simulink model "X8_demo"  (R2015b)
settings: Solver=ode45  StartTime=0.0  StopTime=150  RelTol=1e-3
values from neighbouring files (symbols this model uses):
  end_time = 150    [initX8_demo.m]
  h_ref = 100    [init.m]    (also in initX8_demo.m)
  input_source = 3    [initX8_demo.m]    (also in runX8.m)
  input_source0 = 1    [initX8_demo.m]    (also in runX8.m)
  input_step_time = 0    [initX8_demo.m]    (also in runX8.m = 2)
  lat0 = 37.6205    [init.m]    (also in initX8_demo.m)
  lon0 = -122.3815    [init.m]    (also in initX8_demo.m)
  U_trim = [0.0079    0.0000         0    0.1240]'    [initX8_demo.m]    (also in runX8.m = [0.0079    0.0000         0    0.1240])
  X_trim = [0.0000    0.0000 -150.0000    0.9997    0.0000    0.0232   -0.0000 18.0168    0.0001    0.8366    0.0000    0.0000    0.0000 0.0039 -0.0000    0.0039   -0.0000    0.1240]'    [initX8_demo.m]    (also in runX8.m = x0)
undefined symbols (not defined in the file or in its folder): Earth, WGS84
libraries: simulink x9, simulink_extras x7, aerolibfltsims x4, X8_lib x3, aerolibanimutils x2, aerolibtransform2 x1
settings Model: Creator=krisgry  LastModifiedBy=krisgry
settings DataIOCC: SaveFormat=Array
settings HardwareCC: ProdBitPerPointer=32  ProdLargestAtomicFloat=None  ProdIntDivRoundTo=Undefined  ProdEndianess=Unspecified  ProdWordSize=32  ProdHWDeviceType=32-bit Generic
settings GRTTargetCC: GeneratePreprocessorConditionals=Disable all
settings ConfigComp: CovModelRefEnable=Off

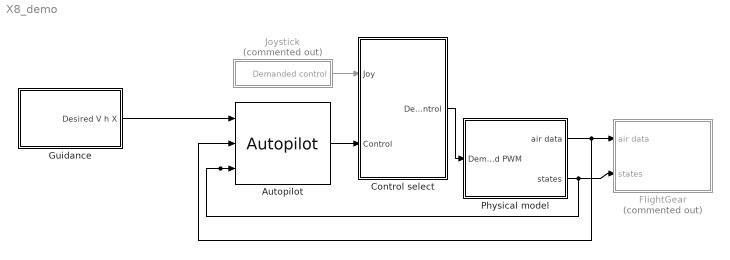
== system X8_demo ==
  Autopilot : X8_lib/Autopilot  param=param  X_trim=X_trim  U_trim=U_trim
  Control select : Subsystem
  FlightGear : Subsystem  Commented=on
  Guidance : Subsystem
  Joystick : Subsystem  Commented=on
  Physical model : Subsystem
  wires:
  Physical model/1(air data) -> Autopilot/2, FlightGear/1(air data)
  Joystick/1(Demanded control) -> Control select/1(Joy)
  Control select/1(Demanded control) -> Physical model/1(Demanded PWM)
  Autopilot/1 -> Control select/2(Control)
  Guidance/1(Desired V h X) -> Autopilot/1
  Physical model/2(states) -> Autopilot/3, FlightGear/2(states)

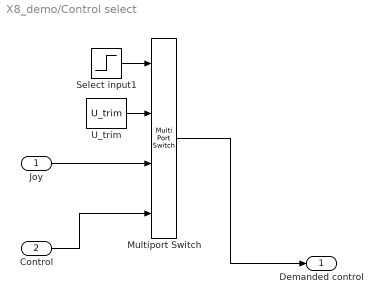
== system X8_demo/Control select ==
  Joy : Inport
  Control : Inport  Port=2
  Multiport Switch : MultiPortSwitch
  Select input1 : Step  Time=input_step_time  Before=input_source0  After=input_source  SampleTime=0
  U_trim : Constant  Value=U_trim
  Demanded control : Outport
  wires:
  Control/1 -> Multiport Switch/4
  Multiport Switch/1 -> Demanded control/1
  U_trim/1 -> Multiport Switch/2
  Joy/1 -> Multiport Switch/3
  Select input1/1 -> Multiport Switch/1

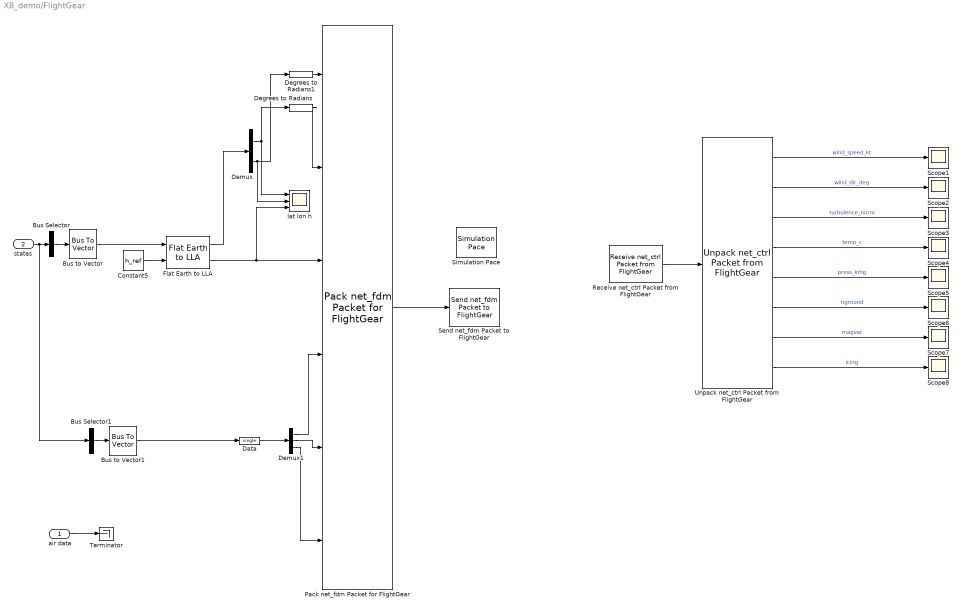
== system X8_demo/FlightGear ==
  air data : Inport
  states : Inport  Port=2
  Bus Selector : BusSelector  OutputSignals=Position.p_N,Position.p_E,Position.p_D  OutputAsBus=on
  Bus Selector1 : BusSelector  OutputSignals=Attitude  OutputAsBus=on
  Bus to Vector : BusToVector
  Bus to Vector1 : BusToVector
  Constant5 : Constant  Value=h_ref
  Data : DataTypeConversion  OutDataTypeStr=single
  Degrees to Radians : simulink_extras/Transformations/Degrees to Radians
  Degrees to Radians1 : simulink_extras/Transformations/Degrees to Radians
  Demux : Demux  Outputs=2
  Demux1 : Demux  Outputs=3
  Flat Earth to LLA : aerolibtransform2/Flat Earth to LLA  units=Metric (MKS)  ptype=Earth (WGS84)  F=1/298.257223563  R=6378137  LL0=[lat0 lon0]  psi=0
  Pack net_fdm Packet for FlightGear : aerolibfltsims/Pack net_fdm Packet for FlightGear  FlightGearVersion=v2.12  ShowPositionAttitudeInputs=on  ShowVelocityAccelerationInputs=off  ShowControlSurfacePositionInputs=off  ShowEngineFuelInputs=off  ShowLandingGearInputs=off  ShowEnvironmentInputs=off  SampleTime=1/30
  Receive net_ctrl Packet from FlightGear : aerolibfltsims/Receive net_ctrl Packet from FlightGear  FlightGearVersion=v2.12  ReceiveAddress=129.241.154.119  ReceivePort=5505  ReceiveWidth=744  varLen=off  SampleTime=1/30  packetFlag=off
      settings: AttributesFormatString=Version Selected:\n%<FlightGearVersion>
  Scope{1..8} (8 alike) : Scope
  Send net_fdm Packet to FlightGear : aerolibfltsims/Send net_fdm Packet to FlightGear  DestinationIpAddress=129.241.154.119  DestinationPort=5502  LocalIpPort=-1  varLen=off  SampleTime=1/30
  Simulation Pace : aerolibanimutils/Simulation Pace  SimulationPace=1  SleepMode=MATLAB Thread  OutputPaceError=off  SampleTime=1/30
      settings: AttributesFormatString=%<SimulationPace> sec/sec
  Terminator : Terminator
  Unpack net_ctrl Packet from FlightGear : aerolibfltsims/Unpack net_ctrl Packet from FlightGear  FlightGearVersion=v2.12  ShowControlSurfacePositionOutputs=off  ShowEngineFuelOutputs=off  ShowLandingGearOutputs=off  ShowAvionicOutputs=off  ShowEnvironmentOutputs=on  SampleTime=1/30
      settings: AttributesFormatString=Version Selected: %<FlightGearVersion>
  lat lon h : Scope  NumInputPorts=3
  wires:
  Pack net_fdm Packet for FlightGear/1 -> Send net_fdm Packet to FlightGear/1
  Demux1/1 -> Pack net_fdm Packet for FlightGear/4
  Demux1/2 -> Pack net_fdm Packet for FlightGear/5
  Demux1/3 -> Pack net_fdm Packet for FlightGear/6
  Demux/2 -> lat lon h/2, Degrees to Radians1/1
  Demux/1 -> Degrees to Radians/1, lat lon h/1
  Data/1 -> Demux1/1
  Degrees to Radians/1 -> Pack net_fdm Packet for FlightGear/2
  Degrees to Radians1/1 -> Pack net_fdm Packet for FlightGear/1
  Unpack net_ctrl Packet from FlightGear/1 -> Scope1/1  "wind_speed_kt"
  Receive net_ctrl Packet from FlightGear/1 -> Unpack net_ctrl Packet from FlightGear/1
  Unpack net_ctrl Packet from FlightGear/2 -> Scope2/1  "wind_dir_deg"
  Unpack net_ctrl Packet from FlightGear/3 -> Scope3/1  "turbulence_norm"
  Unpack net_ctrl Packet from FlightGear/4 -> Scope4/1  "temp_c"
  Unpack net_ctrl Packet from FlightGear/5 -> Scope5/1  "press_inhg"
  Unpack net_ctrl Packet from FlightGear/6 -> Scope6/1  "hground"
  Unpack net_ctrl Packet from FlightGear/7 -> Scope7/1  "magvar"
  Unpack net_ctrl Packet from FlightGear/8 -> Scope8/1  "icing"
  air data/1 -> Terminator/1
  Constant5/1 -> Flat Earth to LLA/2
  Flat Earth to LLA/1 -> Demux/1
  Bus Selector/1 -> Bus to Vector/1
  Bus to Vector/1 -> Flat Earth to LLA/1
  Flat Earth to LLA/2 -> lat lon h/3, Pack net_fdm Packet for FlightGear/3
  Bus Selector1/1 -> Bus to Vector1/1
  Bus to Vector1/1 -> Data/1
  states/1 -> Bus Selector1/1, Bus Selector/1

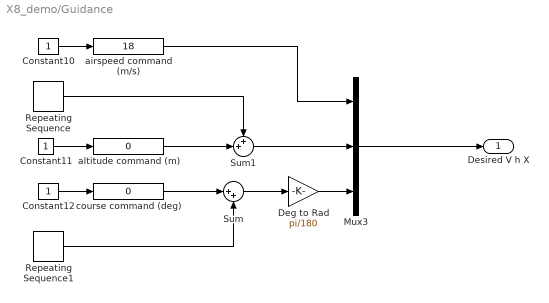
== system X8_demo/Guidance ==
  Constant10 : Constant
  Constant11 : Constant
  Constant12 : Constant
  Deg to Rad : Gain  Gain=pi/180
  Mux3 : Mux  Inputs=3
  Repeating Sequence : simulink/Sources/Repeating Sequence  rep_seq_t=[0 30 70 100 end_time]  rep_seq_y=[150 150 100 100 100]
  Repeating Sequence1 : simulink/Sources/Repeating Sequence  rep_seq_t=[0 70 100 end_time]  rep_seq_y=[0 0 45 45]
  Sum : Sum  Inputs=|++
  Sum1 : Sum  Inputs=++|
  airspeed command (m/s) : simulink/Math Operations/Slider Gain  low=5  gain=18  high=20
  altitude command (m) : simulink/Math Operations/Slider Gain  low=0  gain=0  high=500
  course command (deg) : simulink/Math Operations/Slider Gain  low=-360  gain=0  high=360
  Desired V h X : Outport
  wires:
  Constant12/1 -> course command (deg)/1
  airspeed command (m/s)/1 -> Mux3/1
  Constant10/1 -> airspeed command (m/s)/1
  Constant11/1 -> altitude command (m)/1
  course command (deg)/1 -> Sum/1
  Mux3/1 -> Desired V h X/1
  altitude command (m)/1 -> Sum1/2
  Repeating Sequence1/1 -> Sum/2
  Deg to Rad/1 -> Mux3/3
  Repeating Sequence/1 -> Sum1/1
  Sum1/1 -> Mux3/2
  Sum/1 -> Deg to Rad/1

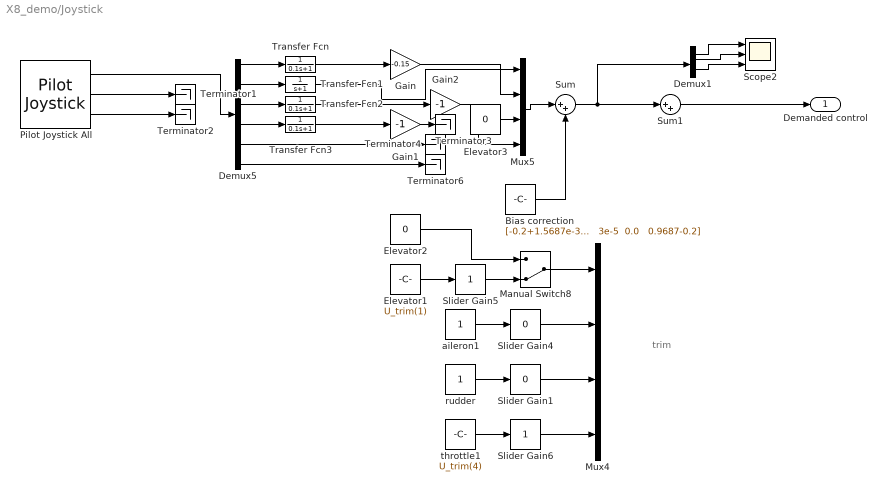
== system X8_demo/Joystick ==
  note: trim
  Bias correction : Constant  Value="[-0.2+1.5687e-3   3e-5  0.0   0.9687-0.2]"
  Demux1 : Demux
  Demux5 : Demux  Outputs=6
  Elevator1 : Constant  Value=U_trim(1)
  Elevator2 : Constant  Value=0
  Elevator3 : Constant  Value=0
  Gain : Gain  Gain=-0.15
  Gain1 : Gain  Gain=-1
  Gain2 : Gain  Gain=-1
  Manual Switch8 : ManualSwitch  CurrentSetting=0
  Mux4 : Mux
  Mux5 : Mux
  Pilot Joystick All : aerolibanimutils/Pilot Joystick  JoystickID=Joystick1  OutputConfiguration=AllOutputs  SampleTime=1/30
  Scope2 : Scope  NumInputPorts=3
  Slider Gain1 : simulink/Math Operations/Slider Gain  low=-1  gain=0  high=1
  Slider Gain4 : simulink/Math Operations/Slider Gain  low=-1  gain=0  high=1
  Slider Gain5 : simulink/Math Operations/Slider Gain  low=-1  gain=1  high=1
  Slider Gain6 : simulink/Math Operations/Slider Gain  low=0  gain=1  high=2
  Sum : Sum  Inputs=|++
  Sum1 : Sum  Inputs=|++
  Terminator{1..4,6} (5 alike) : Terminator
  Transfer Fcn : TransferFcn  Denominator=[0.1 1]
  Transfer Fcn1 : TransferFcn  Denominator=[1 1]
  Transfer Fcn2 : TransferFcn  Denominator=[0.1 1]
  Transfer Fcn3 : TransferFcn  Denominator=[0.1 1]
  aileron1 : Constant
  rudder : Constant
  throttle1 : Constant  Value=U_trim(4)
  Demanded control : Outport
  wires:
  Gain/1 -> Mux5/2
  Demux5/5 -> Terminator4/1
  Demux5/1 -> Transfer Fcn/1
  Demux5/6 -> Terminator6/1
  Demux5/4 -> Transfer Fcn3/1
  Pilot Joystick All/3 -> Terminator2/1
  Pilot Joystick All/2 -> Terminator1/1
  Gain1/1 -> Terminator3/1
  Demux5/3 -> Transfer Fcn2/1
  Mux5/1 -> Sum/1
  Bias correction/1 -> Sum/2
  Gain2/1 -> Mux5/4
  Demux1/1 -> Scope2/1
  Demux1/2 -> Scope2/2
  Sum/1 -> Sum1/1, Demux1/1
  Elevator1/1 -> Slider Gain5/1
  aileron1/1 -> Slider Gain4/1
  Slider Gain4/1 -> Mux4/2
  Slider Gain6/1 -> Mux4/4
  Manual Switch8/1 -> Mux4/1
  Slider Gain5/1 -> Manual Switch8/2
  Elevator2/1 -> Manual Switch8/1
  Sum1/1 -> Demanded control/1
  throttle1/1 -> Slider Gain6/1
  Demux1/4 -> Scope2/3
  Elevator3/1 -> Mux5/3
  rudder/1 -> Slider Gain1/1
  Slider Gain1/1 -> Mux4/3
  Demux5/2 -> Transfer Fcn1/1
  Pilot Joystick All/1 -> Demux5/1
  Transfer Fcn/1 -> Gain/1
  Transfer Fcn1/1 -> Mux5/1
  Transfer Fcn2/1 -> Gain2/1
  Transfer Fcn3/1 -> Gain1/1

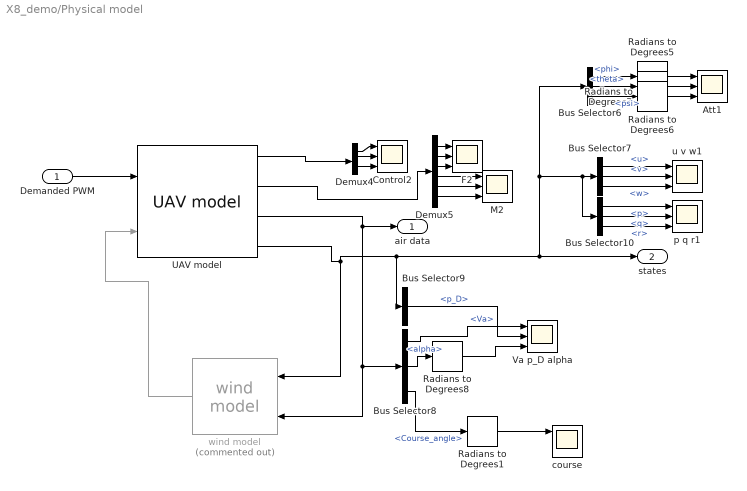
== system X8_demo/Physical model ==
  Demanded PWM : Inport
  Att1 : Scope  NumInputPorts=3
  Bus Selector10 : BusSelector  OutputSignals=AngularVelocity.p,AngularVelocity.q,AngularVelocity.r
  Bus Selector6 : BusSelector  OutputSignals=Attitude.phi,Attitude.theta,Attitude.psi
  Bus Selector7 : BusSelector  OutputSignals=Velocity.u,Velocity.v,Velocity.w
  Bus Selector8 : BusSelector  OutputSignals=Va,alpha,Course_angle
  Bus Selector9 : BusSelector  OutputSignals=Position.p_D
  Control2 : Scope  NumInputPorts=3
  Demux4 : Demux
  Demux5 : Demux  Outputs=6
  F2 : Scope  NumInputPorts=3
  M2 : Scope  NumInputPorts=3
  Radians to Degrees{1,5..8} (5 alike) : simulink_extras/Transformations/Radians to Degrees
  UAV model : X8_lib/UAV model  param=param  pos0=X_trim(1:3)'  quat0=X_trim(4:7)'  vel0=X_trim(8:10)'  rate0=X_trim(11:13)'  servoR_pos0=X_trim(14)  servoR_vel0=X_trim(15)  servoL_pos0=X_trim(16)  servoL_vel0=X_trim(17)  motor_speed0=X_trim(18)
  Va p_D alpha : Scope  NumInputPorts=3
  course : Scope  NumInputPorts=3
  p q r1 : Scope  NumInputPorts=3
  u v w1 : Scope  NumInputPorts=3
  wind model : X8_lib/wind model  Commented=on  wind_speed=0  wind_dir=0  wind_start_time=0  param='x8_param'
  air data : Outport
  states : Outport  Port=2
  wires:
  Demux5/1 -> F2/1
  Demux5/2 -> F2/2
  Demux5/3 -> F2/3
  Demux5/4 -> M2/1
  Demux5/5 -> M2/2
  Demux5/6 -> M2/3
  Bus Selector7/1 -> u v w1/1  "<u>"
  Bus Selector7/2 -> u v w1/2  "<v>"
  Bus Selector7/3 -> u v w1/3  "<w>"
  Bus Selector6/1 -> Radians to Degrees5/1  "<phi>"
  Bus Selector6/3 -> Radians to Degrees7/1  "<psi>"
  Bus Selector6/2 -> Radians to Degrees6/1  "<theta>"
  Radians to Degrees5/1 -> Att1/1
  Radians to Degrees6/1 -> Att1/2
  Radians to Degrees7/1 -> Att1/3
  Bus Selector8/1 -> Va p_D alpha/1  "<Va>"
  Bus Selector9/1 -> Va p_D alpha/2  "<p_D>"
  Bus Selector8/2 -> Radians to Degrees8/1  "<alpha>"
  Radians to Degrees8/1 -> Va p_D alpha/3
  Demux4/4 -> Control2/3
  Demux4/2 -> Control2/2
  Demux4/1 -> Control2/1
  Bus Selector10/1 -> p q r1/1  "<p>"
  Bus Selector10/2 -> p q r1/2  "<q>"
  Bus Selector10/3 -> p q r1/3  "<r>"
  UAV model/3 -> air data/1, wind model/2, Bus Selector8/1
  UAV model/4 -> wind model/1, Bus Selector9/1, Bus Selector6/1, Bus Selector7/1, Bus Selector10/1, states/1
  UAV model/2 -> Demux5/1
  UAV model/1 -> Demux4/1
  wind model/1 -> UAV model/2
  Demanded PWM/1 -> UAV model/1
  Bus Selector8/3 -> Radians to Degrees1/1  "<Course_angle>"
  Radians to Degrees1/1 -> course/1
